simulink model "L6_sim2"  (R2024b)
settings: Solver=VariableStepAuto  StartTime=0.0  StopTime=100  RelTol=1e-3
values from neighbouring files (symbols this model uses):
  A_0 = eye(3)    [Task2.m]
  G = 6.673e-20    [Task2.m]
  I = diag([Ix, Iy, Iz])    [Task1.m]    (also in Task2.m = diag([Ix(3), Iy(3), Iz(3)]))
  M_t = 5.973e24    (= 5.973e+24)    [Task2.m]
  n = sqrt(G*M_t/R^3)    [Task2.m]
  orthonormalize = 0    [Task2.m]
  R = Rt+H    (= 6878.137)    [Task2.m]
  w_0 = [0.3, 0.15, 0.6]'    [Task1.m]    (also in Task2.m = [1e-6, n, 1e-6]')
libraries: matrix_library x2
settings Model: Creator=alejandromunozvazquez  LastModifiedBy=alejandromunozvazquez

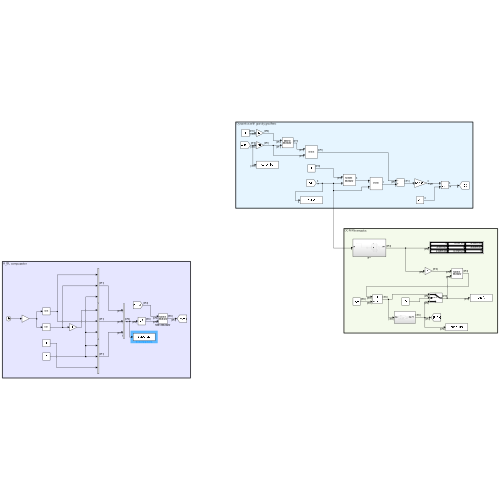
[thumbnail: Simulink's stored preview of the top-level diagram]
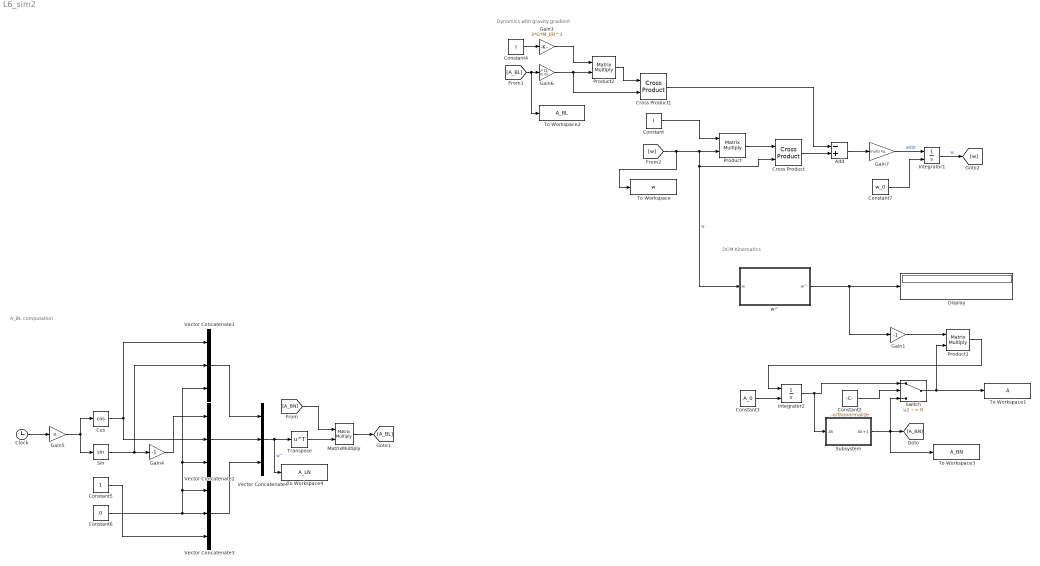
== system L6_sim2 ==
  note: Dynamics with gravity gradient
  note: DCM Kinematics
  note: A_BL computation
  Add : Sum  Inputs=-+
  Clock : Clock
  Constant : Constant  Value=I
  Constant2 : Constant  Value=-orthonormalize
  Constant3 : Constant  Value=A_0
  Constant4 : Constant  Value=I
  Constant5 : Constant
  Constant6 : Constant  Value=0
  Constant7 : Constant  Value=w_0
  Cos : Trigonometry  Operator=cos
  Cross Product : matrix_library/Cross Product
  Cross Product1 : matrix_library/Cross Product
  Display : Display
  Gain1 : Gain  Gain=-1
  Gain3 : Gain  Gain=3*G*M_t/R^3
  Gain4 : Gain  Gain=-1
  Gain5 : Gain  Gain=n
  Gain6 : Gain  Gain=[1; 0; 0]  Multiplication=Matrix(u*K)
  Gain7 : Gain  Gain=inv(I)  Multiplication=Matrix(K*u) (u vector)
  Integrator1 : Integrator  InitialConditionSource=external
  Integrator2 : Integrator  InitialConditionSource=external
  MatrixMultiply : Product  Multiplication=Matrix(*)
  Product : Product  Multiplication=Matrix(*)
  Product1 : Product  Multiplication=Matrix(*)
  Product2 : Product  Multiplication=Matrix(*)
  Sin : Trigonometry
  Subsystem : Subsystem
  Switch : Switch  Criteria=u2 ~= 0  SaturateOnIntegerOverflow=off  InputSameDT=off
  To Workspace : ToWorkspace  VariableName=w  SampleTime=-1
  To Workspace1 : ToWorkspace  VariableName=A  SampleTime=-1
  To Workspace2 : ToWorkspace  VariableName=A_BL  SampleTime=-1
  To Workspace3 : ToWorkspace  VariableName=A_BN  SampleTime=-1
  To Workspace4 : ToWorkspace  VariableName=A_LN  SampleTime=-1
  Transpose : Math  Operator=transpose
  Vector Concatenate1 : Concatenate  NumInputs=3  Mode=Multidimensional array
  Vector Concatenate2 : Concatenate  NumInputs=3  Mode=Multidimensional array
  Vector Concatenate3 : Concatenate  NumInputs=3  Mode=Multidimensional array
  Vector Concatenate4 : Concatenate  NumInputs=3  Mode=Multidimensional array  ConcatenateDimension=2
  "w^ " : Subsystem
  wires:
  [w] -> Cross Product/2, "w^ "/1(w), Product/2, To Workspace/1  "w"
  Constant/1 -> Product/1
  Product/1 -> Cross Product/1
  Cross Product/1 -> Add/2
  Product1/1 -> Integrator2/1
  Constant3/1 -> Integrator2/2
  Gain1/1 -> Product1/1
  Switch/1 -> Product1/2, To Workspace1/1
  "w^ "/1(w^) -> Gain1/1, Display/1
  Integrator2/1 -> Subsystem/1(Ak), Switch/1
  Subsystem/1(Ak+1) -> To Workspace3/1, [A_BN], Switch/3
  Constant2/1 -> Switch/2
  Product2/1 -> Cross Product1/1
  Constant4/1 -> Gain3/1
  Gain3/1 -> Product2/1
  Gain6/1 -> Cross Product1/2, Product2/2
  [A_BL] -> To Workspace2/1, Gain6/1
  Add/1 -> Gain7/1
  Cross Product1/1 -> Add/1
  Gain7/1 -> Integrator1/1  "wdot"
  Constant7/1 -> Integrator1/2
  Integrator1/1 -> [w]  "w"
  Constant6/1 -> Vector Concatenate3/2, Vector Concatenate3/1, Vector Concatenate2/3, Vector Concatenate1/3
  MatrixMultiply/1 -> [A_BL]
  Constant5/1 -> Vector Concatenate3/3
  Gain4/1 -> Vector Concatenate2/1
  [A_BN] -> MatrixMultiply/1
  Vector Concatenate1/1 -> Vector Concatenate4/1
  Vector Concatenate3/1 -> Vector Concatenate4/3
  Vector Concatenate2/1 -> Vector Concatenate4/2
  Gain5/1 -> Sin/1, Cos/1
  Sin/1 -> Gain4/1, Vector Concatenate1/2
  Cos/1 -> Vector Concatenate2/2, Vector Concatenate1/1
  Transpose/1 -> MatrixMultiply/2
  Clock/1 -> Gain5/1
  Vector Concatenate4/1 -> To Workspace4/1, Transpose/1  "w^"

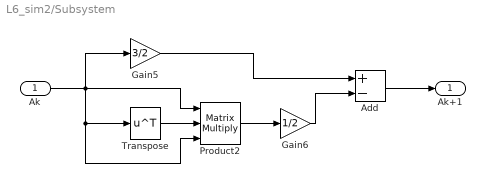
== system L6_sim2/Subsystem ==
  Ak : Inport
  Add : Sum  Inputs=+-
  Gain5 : Gain  Gain=3/2
  Gain6 : Gain  Gain=1/2
  Product2 : Product  Inputs=3  Multiplication=Matrix(*)
  Transpose : Math  Operator=transpose
  Ak+1 : Outport
  wires:
  Gain5/1 -> Add/1
  Add/1 -> Ak+1/1
  Product2/1 -> Gain6/1
  Gain6/1 -> Add/2
  Transpose/1 -> Product2/2
  Ak/1 -> Product2/3, Transpose/1, Gain5/1, Product2/1

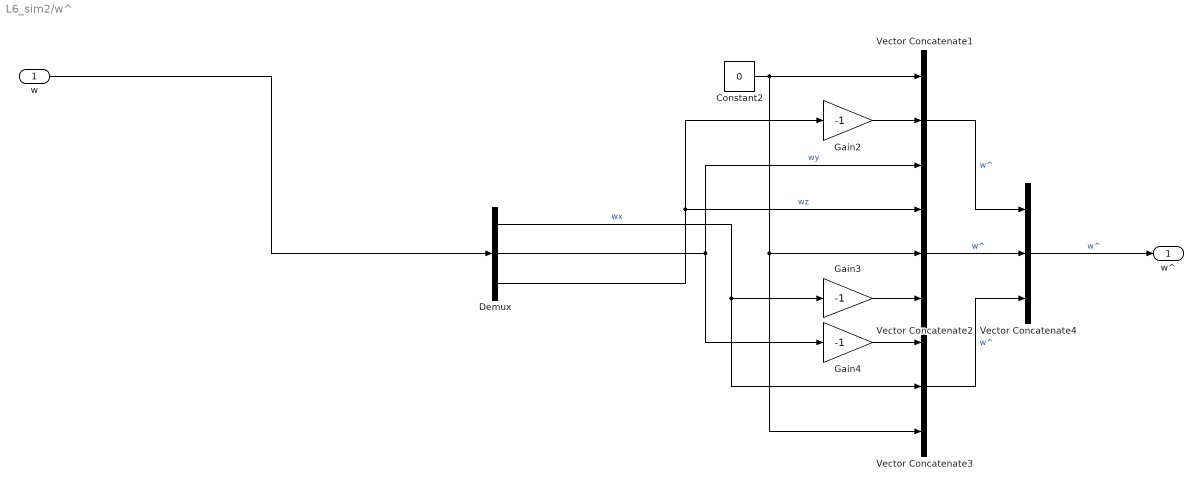
== system L6_sim2/w^  ==
  w : Inport
  Constant2 : Constant  Value=0
  Demux : Demux  Outputs=3
  Gain2 : Gain  Gain=-1
  Gain3 : Gain  Gain=-1
  Gain4 : Gain  Gain=-1
  Vector Concatenate1 : Concatenate  NumInputs=3  Mode=Multidimensional array
  Vector Concatenate2 : Concatenate  NumInputs=3  Mode=Multidimensional array
  Vector Concatenate3 : Concatenate  NumInputs=3  Mode=Multidimensional array
  Vector Concatenate4 : Concatenate  NumInputs=3  Mode=Multidimensional array  ConcatenateDimension=2
  w^ : Outport
  wires:
  w/1 -> Demux/1
  Vector Concatenate4/1 -> w^/1  "w^"
  Demux/2 -> Vector Concatenate1/3, Gain4/1  "wy"
  Vector Concatenate1/1 -> Vector Concatenate4/1  "w^"
  Demux/1 -> Vector Concatenate3/2, Gain3/1  "wx"
  Gain2/1 -> Vector Concatenate1/2
  Vector Concatenate3/1 -> Vector Concatenate4/3  "w^"
  Gain4/1 -> Vector Concatenate3/1
  Constant2/1 -> Vector Concatenate1/1, Vector Concatenate2/2, Vector Concatenate3/3
  Vector Concatenate2/1 -> Vector Concatenate4/2  "w^"
  Gain3/1 -> Vector Concatenate2/3
  Demux/3 -> Gain2/1, Vector Concatenate2/1  "wz"
